simulink model "p2_3p_pll_cosim"  (Simulink 6.4)
settings: Solver=FixedStepDiscrete  SolverMode=SingleTasking  StartTime=0.0  StopTime=0.4  RelTol=1e-3
undefined symbols (not defined in the file or in its folder): pipeline_prec
libraries: modelsimlib x1
settings Model: LastModifiedBy=Administrador

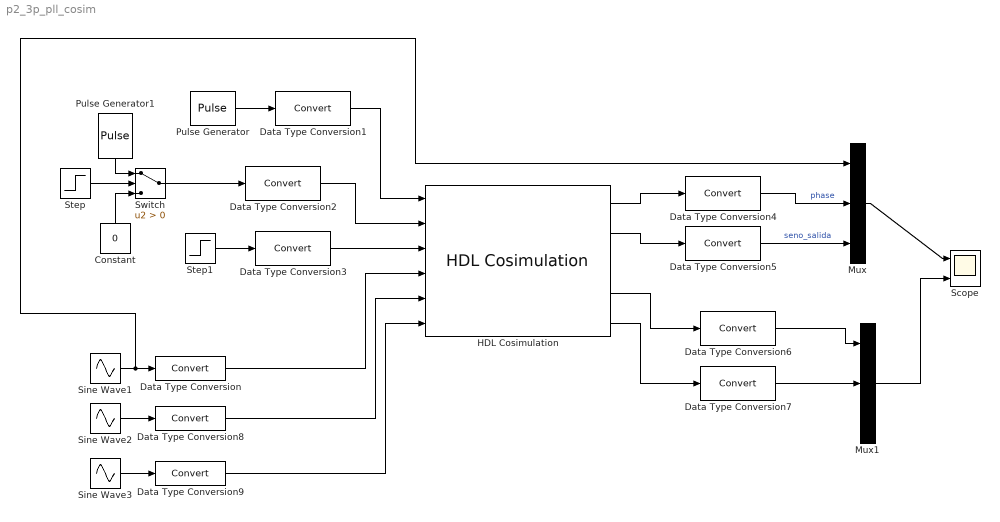
== system p2_3p_pll_cosim ==
  Constant : Constant  Orientation=up  Value=0  OutDataType=sfix(16)  ConRadixGroup=Use specified scaling  OutScaling=2^0  SampleTime=-1  FramePeriod=inf
  Data Type Conversion : DataTypeConversion  OutDataTypeMode=Specify via dialog  OutScaling=2^(-pipeline_prec)  RndMeth=Nearest  SaturateOnIntegerOverflow=on
  Data Type Conversion1 : DataTypeConversion  OutDataTypeMode=boolean
  Data Type Conversion2 : DataTypeConversion  OutDataTypeMode=boolean
  Data Type Conversion3 : DataTypeConversion  OutDataTypeMode=boolean
  Data Type Conversion{4..7} (4 alike) : DataTypeConversion
  Data Type Conversion8 : DataTypeConversion  OutDataTypeMode=Specify via dialog  OutScaling=2^(-pipeline_prec)  RndMeth=Nearest  SaturateOnIntegerOverflow=on
  Data Type Conversion9 : DataTypeConversion  OutDataTypeMode=Specify via dialog  OutScaling=2^(-pipeline_prec)  RndMeth=Nearest  SaturateOnIntegerOverflow=on
  HDL Cosimulation : modelsimlib/HDL Cosimulation  DialogController=modelsimddg.CoSim  DialogControllerArgs=DataTag0  PortPaths=/p2_3p_pll/clk;/p2_3p_pll/sample;/p2_3p_pll/rst;/p2_3p_pll/a;/p2_3p_pll/b;/p2_3p_pll/c;/p2_3p_pll/phase;/p2_3p_pll/ampl;/p2_3p_pll/done;/p2_3p_pll/d_s;/p2_3p_pll/q_s  PortModes=[1 1 1 1 1 1 2 2 2 2 2 ]  PortTimes=[1,1,1,1,1,1,1e-5,1e-5,1,1e-5,1e-5]  PortSigns=[-1 -1 -1 -1 -1 -1 1 1 -1 1 1 ]  PortFracLengths=[0,0,0,0,0,0,pipeline_prec,pipeline_prec,pipeline_prec,pipeline_prec,pipeline_prec]  CommLocal=on  CommSharedMemory=off  CommPortNumber=4449  CommShowInfo=on  ClockModes=[]  ClockTimes=[]  TclPreSimCommand="echo \"Running Simulink Cosimulation block.\""  TclPostSimCommand="echo \"done\""  TimingMode=s  TimingScaleFactor=1  idxCellArray={'UNUSED_VAR'}
  Mux : Mux  Inputs=3
  Mux1 : Mux  Inputs=3
  Pulse Generator : DiscretePulseGenerator  PulseType=Time based  Period=1/(1e6)  PulseWidth=50
  Pulse Generator1 : DiscretePulseGenerator  Orientation=down  PulseType=Time based  Period=0.1e-3  PulseWidth=2
  Scope : Scope  NumInputPorts=2
      settings: YMin=-3.5~-0.05  YMax=3.5~1  MaxDataPoints=500000
  Sine Wave1 : Sin  Frequency=2*pi*50.5
  Sine Wave2 : Sin  Frequency=2*pi*50.5  Phase=-2*pi/3
  Sine Wave3 : Sin  Frequency=2*pi*50.5  Phase=2*pi/3
  Step : Step  Time=4*(1/1e6)
  Step1 : Step  Time=6*(1/1e6)  Before=1  After=0
  Switch : Switch  Criteria=u2 > Threshold  RndMeth=Nearest  ZeroCross=off  SampleTime=1e-7
  wires:
  Pulse Generator/1 -> Data Type Conversion1/1
  Data Type Conversion1/1 -> HDL Cosimulation/1
  Switch/1 -> Data Type Conversion2/1
  Data Type Conversion2/1 -> HDL Cosimulation/2
  Step1/1 -> Data Type Conversion3/1
  Data Type Conversion3/1 -> HDL Cosimulation/3
  Constant/1 -> Switch/3
  Step/1 -> Switch/2
  Mux/1 -> Scope/1
  HDL Cosimulation/1 -> Data Type Conversion4/1
  Data Type Conversion4/1 -> Mux/2  "phase"
  Data Type Conversion5/1 -> Mux/3  "seno_salida"
  HDL Cosimulation/2 -> Data Type Conversion5/1
  Data Type Conversion6/1 -> Mux1/1
  Data Type Conversion7/1 -> Mux1/2
  Mux1/1 -> Scope/2
  Sine Wave1/1 -> Data Type Conversion/1, Mux/1
  Sine Wave2/1 -> Data Type Conversion8/1
  Sine Wave3/1 -> Data Type Conversion9/1
  Data Type Conversion/1 -> HDL Cosimulation/4
  Data Type Conversion8/1 -> HDL Cosimulation/5
  Data Type Conversion9/1 -> HDL Cosimulation/6
  Pulse Generator1/1 -> Switch/1
  HDL Cosimulation/4 -> Data Type Conversion6/1
  HDL Cosimulation/5 -> Data Type Conversion7/1
